simulink model "P702_NI_SoftECU"  (R2019a)
settings: Solver=ode1  StartTime=0.0  StopTime=Inf  FixedStep=0.001  RelTol=1e-3  EnableMultiTasking=on
PreLoadFcn:
  | run '.\VeriStand_BlockSet\NIVeriStandAddPaths.m'
undefined symbols (not defined in the file or in its folder): magnitude
libraries: simulink x83, simulink_extras x1
(part 18 of 76)

== system P702_NI_SoftECU/Input/ECM_DIESEL PCM PCM_HEV/PowertrainData_1_0x421 ==
  AirCondFluidHi_P_Actl : Constant  Commented=on  Value=0
  Bus_Sig : BusCreator  Inputs=12
  CoolantFanStepAct : Constant  Commented=on  Value=0
  ECMMILRequest : Constant  Commented=on  Value=0
  EngIdlShutDown_D_Stat : Constant  Commented=on  Value=0
  EngIdlShutDwnTxt_D_Rq : Constant  Commented=on  Value=0
  FUEL_ALCOHOL_PERCNT : Constant  Commented=on  Value=100.393700685
  FohEng_D_Rq : Constant  Commented=on  Value=2
  OilPressureWarning : Constant  Commented=on  Value=0
  TrnTotLss_Tq_Est : Constant  Commented=on  Value=0
  TrnTotTq_Rt_Est : Constant  Commented=on  Value=0
  VehVLimActv_B_Actl : Constant  Commented=on  Value=0
  VehVLimStat_D_Actl : Constant  Commented=on  Value=0
  PowertrainData_1_0x421 : Outport
  wires:
  Bus_Sig/1 -> PowertrainData_1_0x421/1  "PowertrainData_1_0x421"
  VehVLimActv_B_Actl/1 -> Bus_Sig/1  "VehVLimActv_B_Actl"
  VehVLimStat_D_Actl/1 -> Bus_Sig/2  "VehVLimStat_D_Actl"
  ECMMILRequest/1 -> Bus_Sig/3  "ECMMILRequest"
  FohEng_D_Rq/1 -> Bus_Sig/4  "FohEng_D_Rq"
  EngIdlShutDown_D_Stat/1 -> Bus_Sig/5  "EngIdlShutDown_D_Stat"
  CoolantFanStepAct/1 -> Bus_Sig/6  "CoolantFanStepAct"
  OilPressureWarning/1 -> Bus_Sig/7  "OilPressureWarning"
  EngIdlShutDwnTxt_D_Rq/1 -> Bus_Sig/8  "EngIdlShutDwnTxt_D_Rq"
  TrnTotLss_Tq_Est/1 -> Bus_Sig/9  "TrnTotLss_Tq_Est"
  TrnTotTq_Rt_Est/1 -> Bus_Sig/10  "TrnTotTq_Rt_Est"
  AirCondFluidHi_P_Actl/1 -> Bus_Sig/11  "AirCondFluidHi_P_Actl"
  FUEL_ALCOHOL_PERCNT/1 -> Bus_Sig/12  "FUEL_ALCOHOL_PERCNT"

== system P702_NI_SoftECU/Input/ECM_DIESEL PCM PCM_HEV/PowertrainData_2_0x42D ==
  ApedPos_Pc_ActlDiag : Constant  Commented=on  Value=0
  Bus_Sig : BusCreator  Inputs=11
  EngAirIn_Te_Actl : Constant  Commented=on  Value=-128
  EngClnt_Te_ActlDiag : Constant  Commented=on  Value=-40
  EngLoad_Pc_CalcDiag : Constant  Commented=on  Value=0
  EngMsgTxt_D_Rq : Constant  Commented=on  Value=0
  GrllShtrPos_B_Falt : Constant  Commented=on  Value=0
  GrllShtrPos_D_Cmd : Constant  Commented=on  Value=0
  IsaOffst_D_Stat : Constant  Commented=on  Value=0
  ObdWarmUp_B_Complt : Constant  Commented=on  Value=0
  SlMde_D_RqDsply : Constant  Commented=on  Value=0
  SlMde_D_Stat : Constant  Commented=on  Value=0
  PowertrainData_2_0x42D : Outport
  wires:
  Bus_Sig/1 -> PowertrainData_2_0x42D/1  "PowertrainData_2_0x42D"
  ObdWarmUp_B_Complt/1 -> Bus_Sig/1  "ObdWarmUp_B_Complt"
  EngMsgTxt_D_Rq/1 -> Bus_Sig/2  "EngMsgTxt_D_Rq"
  EngAirIn_Te_Actl/1 -> Bus_Sig/3  "EngAirIn_Te_Actl"
  ApedPos_Pc_ActlDiag/1 -> Bus_Sig/4  "ApedPos_Pc_ActlDiag"
  EngClnt_Te_ActlDiag/1 -> Bus_Sig/5  "EngClnt_Te_ActlDiag"
  EngLoad_Pc_CalcDiag/1 -> Bus_Sig/6  "EngLoad_Pc_CalcDiag"
  GrllShtrPos_D_Cmd/1 -> Bus_Sig/7  "GrllShtrPos_D_Cmd"
  GrllShtrPos_B_Falt/1 -> Bus_Sig/8  "GrllShtrPos_B_Falt"
  IsaOffst_D_Stat/1 -> Bus_Sig/9  "IsaOffst_D_Stat"
  SlMde_D_RqDsply/1 -> Bus_Sig/10  "SlMde_D_RqDsply"
  SlMde_D_Stat/1 -> Bus_Sig/11  "SlMde_D_Stat"

== system P702_NI_SoftECU/Input/ECM_DIESEL PCM PCM_HEV/PowertrainData_3_0x43E ==
  BattULoChrg_U_Cmd : Constant  Commented=on  Value=10.6
  Bus_Sig : BusCreator  Inputs=4
  ElLoadCtl_D_Rq : Constant  Commented=on  Value=0
  EngMnfld_P_Actl : Constant  Commented=on  Value=-206.8
  FuelPumpPwr_B_Rq : Constant  Commented=on  Value=0
  PowertrainData_3_0x43E : Outport
  wires:
  Bus_Sig/1 -> PowertrainData_3_0x43E/1  "PowertrainData_3_0x43E"
  BattULoChrg_U_Cmd/1 -> Bus_Sig/1  "BattULoChrg_U_Cmd"
  ElLoadCtl_D_Rq/1 -> Bus_Sig/2  "ElLoadCtl_D_Rq"
  FuelPumpPwr_B_Rq/1 -> Bus_Sig/3  "FuelPumpPwr_B_Rq"
  EngMnfld_P_Actl/1 -> Bus_Sig/4  "EngMnfld_P_Actl"

== system P702_NI_SoftECU/Input/ECM_DIESEL PCM PCM_HEV/PowertrainData_6_0x205 ==
  BrkTot_Tq_RqFapLc : Constant  Commented=on  Value=0
  Bus_Sig : BusCreator  Inputs=3
  FapLc_B_Err : S-Function  Priority=1  FunctionName=NIVeriStandIO  Parameters=width dtype portnum stime stype btype  SFunctionDeploymentMode=off  EnableBusSupport=off  mask(NI VeriStand Inport){portnum=1, width=1, stime=-1, dtype=auto, stype=auto, btype=1}
      mask prompts: portnum "Port number:"; width "Port dimensions (-1 for dynamically sized):"; stime "Sample time (-1 for inherited):"; dtype "Data type:"; stype "Signal type:"; btype "Block type:"
      mask help: Use this inport on any level of nested subsystems to allow NI VeriStand software to map signals to it.
      mask init:
      | NIVeriStandIO_init;
      settings: CopyFcn=NIVeriStand_MDL_functions('', 'IO_copy');  DeleteFcn=NIVeriStand_MDL_functions('', 'IO_delete');  MoveFcn=set_param(gcb, 'Mask', 'on');
      mask Callback portnum: NIVeriStand_MDL_functions('', 'IO_setportnum');
      mask TypeOptions dtype: auto | double | single | int8 | uint8 | int16 | uint16 | int32 | uint32 | boolean
      mask Callback dtype: NIVeriStand_MDL_functions('', 'IO_booleansignal');
      mask TypeOptions stype: auto | real | complex
      mask Display:
      | patch([-x x], [-y y], [.90980 .81960 .32156]);
      | plot([xrad -x x xrad], [yrad -y y yrad]);
      | fprintf('NI In%d', portnum);
  TrnAin_Pc_RqDrv : Constant  Commented=on  Value=0
  PowertrainData_6_0x205 : Outport
  wires:
  Bus_Sig/1 -> PowertrainData_6_0x205/1  "PowertrainData_6_0x205"
  BrkTot_Tq_RqFapLc/1 -> Bus_Sig/1  "BrkTot_Tq_RqFapLc"
  FapLc_B_Err/1 -> Bus_Sig/2  "FapLc_B_Err"
  TrnAin_Pc_RqDrv/1 -> Bus_Sig/3  "TrnAin_Pc_RqDrv"

== system P702_NI_SoftECU/Input/ECM_DIESEL PCM PCM_HEV/PowertrainData_7_0x41F ==
  Bus_Sig : BusCreator  Inputs=7
  EcoCochA_Pc_Dsply : Constant  Commented=on  Value=100.000035
  EcoCochCrus_Pc_Dsply : Constant  Commented=on  Value=100.000035
  EcoCochDecel_Pc_Dsply : Constant  Commented=on  Value=100.000035
  EcoCochIdlFuel_Pc_Dsply : Constant  Commented=on  Value=100.000035
  EcoCochInstNeg_B_Dsply : Constant  Commented=on  Value=0
  EcoCochInst_Pc_Dsply : Constant  Commented=on  Value=10
  EcoCochShif_Pc_Dsply : Constant  Commented=on  Value=100.000035
  PowertrainData_7_0x41F : Outport
  wires:
  Bus_Sig/1 -> PowertrainData_7_0x41F/1  "PowertrainData_7_0x41F"
  EcoCochA_Pc_Dsply/1 -> Bus_Sig/1  "EcoCochA_Pc_Dsply"
  EcoCochCrus_Pc_Dsply/1 -> Bus_Sig/2  "EcoCochCrus_Pc_Dsply"
  EcoCochDecel_Pc_Dsply/1 -> Bus_Sig/3  "EcoCochDecel_Pc_Dsply"
  EcoCochIdlFuel_Pc_Dsply/1 -> Bus_Sig/4  "EcoCochIdlFuel_Pc_Dsply"
  EcoCochShif_Pc_Dsply/1 -> Bus_Sig/5  "EcoCochShif_Pc_Dsply"
  EcoCochInst_Pc_Dsply/1 -> Bus_Sig/6  "EcoCochInst_Pc_Dsply"
  EcoCochInstNeg_B_Dsply/1 -> Bus_Sig/7  "EcoCochInstNeg_B_Dsply"

== system P702_NI_SoftECU/Input/ECM_DIESEL PCM PCM_HEV/PowertrainData_9_0x44C ==
  AutoTowActv_B_Stat : Constant  Commented=on  Value=0
  AutoTowAllw_D_StatMnu : Constant  Commented=on  Value=0
  Bus_Sig : BusCreator  Inputs=7
  GrossTrainWeight_M_Est : Constant  Commented=on  Value=25400
  TrailCtlPt_B_Falt : Constant  Commented=on  Value=0
  Veh_V_DsplyTrailCtlSet : Constant  Commented=on  Value=0
  WakeAlarm1_B_Typ : Constant  Commented=on  Value=0
  WakeAlarm1_T_Rq : Constant  Commented=on  Value=32767
  PowertrainData_9_0x44C : Outport
  wires:
  Bus_Sig/1 -> PowertrainData_9_0x44C/1  "PowertrainData_9_0x44C"
  GrossTrainWeight_M_Est/1 -> Bus_Sig/1  "GrossTrainWeight_M_Est"
  AutoTowAllw_D_StatMnu/1 -> Bus_Sig/2  "AutoTowAllw_D_StatMnu"
  AutoTowActv_B_Stat/1 -> Bus_Sig/3  "AutoTowActv_B_Stat"
  TrailCtlPt_B_Falt/1 -> Bus_Sig/4  "TrailCtlPt_B_Falt"
  Veh_V_DsplyTrailCtlSet/1 -> Bus_Sig/5  "Veh_V_DsplyTrailCtlSet"
  WakeAlarm1_T_Rq/1 -> Bus_Sig/6  "WakeAlarm1_T_Rq"
  WakeAlarm1_B_Typ/1 -> Bus_Sig/7  "WakeAlarm1_B_Typ"

== system P702_NI_SoftECU/Input/ECM_DIESEL PCM PCM_HEV/Powertrain_Data_4_0x424 ==
  BpedDrvMsgTxt_B_Dsply : Constant  Commented=on  Value=0
  Bus_Sig : BusCreator  Inputs=7
  FuelLvlWarn_D_ActlEng : Constant  Commented=on  Value=0
  FuelLvl_Pc_DsplyEng : Constant  Commented=on  Value=-5.217408
  FuelRange_L_DsplyEng : Constant  Commented=on  Value=0
  RearDiffOilTeWarn_B_Rq : Constant  Commented=on  Value=0
  RearDiffOil_Te_Actl : Constant  Commented=on  Value=37
  SelDrvMdePt_D_Stat : Constant  Commented=on  Value=0
  Powertrain_Data_4_0x424 : Outport
  wires:
  Bus_Sig/1 -> Powertrain_Data_4_0x424/1  "Powertrain_Data_4_0x424"
  BpedDrvMsgTxt_B_Dsply/1 -> Bus_Sig/1  "BpedDrvMsgTxt_B_Dsply"
  RearDiffOil_Te_Actl/1 -> Bus_Sig/2  "RearDiffOil_Te_Actl"
  RearDiffOilTeWarn_B_Rq/1 -> Bus_Sig/3  "RearDiffOilTeWarn_B_Rq"
  FuelLvlWarn_D_ActlEng/1 -> Bus_Sig/4  "FuelLvlWarn_D_ActlEng"
  SelDrvMdePt_D_Stat/1 -> Bus_Sig/5  "SelDrvMdePt_D_Stat"
  FuelRange_L_DsplyEng/1 -> Bus_Sig/6  "FuelRange_L_DsplyEng"
  FuelLvl_Pc_DsplyEng/1 -> Bus_Sig/7  "FuelLvl_Pc_DsplyEng"

== system P702_NI_SoftECU/Input/ECM_DIESEL PCM PCM_HEV/Powertrain_Data_5_0x43F ==
  Bus_Sig : BusCreator  Inputs=7
  FapLcActv_B_Stat : S-Function  Priority=1  FunctionName=NIVeriStandIO  Parameters=width dtype portnum stime stype btype  SFunctionDeploymentMode=off  EnableBusSupport=off  mask(NI VeriStand Inport){portnum=1, width=1, stime=-1, dtype=auto, stype=auto, btype=1}
      mask prompts: portnum "Port number:"; width "Port dimensions (-1 for dynamically sized):"; stime "Sample time (-1 for inherited):"; dtype "Data type:"; stype "Signal type:"; btype "Block type:"
      mask help: Use this inport on any level of nested subsystems to allow NI VeriStand software to map signals to it.
      mask init:
      | NIVeriStandIO_init;
      settings: CopyFcn=NIVeriStand_MDL_functions('', 'IO_copy');  DeleteFcn=NIVeriStand_MDL_functions('', 'IO_delete');  MoveFcn=set_param(gcb, 'Mask', 'on');
      mask Callback portnum: NIVeriStand_MDL_functions('', 'IO_setportnum');
      mask TypeOptions dtype: auto | double | single | int8 | uint8 | int16 | uint16 | int32 | uint32 | boolean
      mask Callback dtype: NIVeriStand_MDL_functions('', 'IO_booleansignal');
      mask TypeOptions stype: auto | real | complex
      mask Display:
      | patch([-x x], [-y y], [.90980 .81960 .32156]);
      | plot([xrad -x x xrad], [yrad -y y yrad]);
      | fprintf('NI In%d', portnum);
  FapLcInhbt_B_Rq : Constant  Commented=on  Value=0
  FapLcMaxGrdAbrt_B_Stat : S-Function  Priority=2  FunctionName=NIVeriStandIO  Parameters=width dtype portnum stime stype btype  SFunctionDeploymentMode=off  EnableBusSupport=off  mask(NI VeriStand Inport){portnum=2, width=1, stime=-1, dtype=auto, stype=auto, btype=1}
      mask prompts: portnum "Port number:"; width "Port dimensions (-1 for dynamically sized):"; stime "Sample time (-1 for inherited):"; dtype "Data type:"; stype "Signal type:"; btype "Block type:"
      mask help: Use this inport on any level of nested subsystems to allow NI VeriStand software to map signals to it.
      mask init:
      | NIVeriStandIO_init;
      settings: CopyFcn=NIVeriStand_MDL_functions('', 'IO_copy');  DeleteFcn=NIVeriStand_MDL_functions('', 'IO_delete');  MoveFcn=set_param(gcb, 'Mask', 'on');
      mask Callback portnum: NIVeriStand_MDL_functions('', 'IO_setportnum');
      mask TypeOptions dtype: auto | double | single | int8 | uint8 | int16 | uint16 | int32 | uint32 | boolean
      mask Callback dtype: NIVeriStand_MDL_functions('', 'IO_booleansignal');
      mask TypeOptions stype: auto | real | complex
      mask Display:
      | patch([-x x], [-y y], [.90980 .81960 .32156]);
      | plot([xrad -x x xrad], [yrad -y y yrad]);
      | fprintf('NI In%d', portnum);
  FapLcMaxGrdInhbt_B_Stat : S-Function  Priority=3  FunctionName=NIVeriStandIO  Parameters=width dtype portnum stime stype btype  SFunctionDeploymentMode=off  EnableBusSupport=off  mask(NI VeriStand Inport){portnum=3, width=1, stime=-1, dtype=auto, stype=auto, btype=1}
      mask prompts: portnum "Port number:"; width "Port dimensions (-1 for dynamically sized):"; stime "Sample time (-1 for inherited):"; dtype "Data type:"; stype "Signal type:"; btype "Block type:"
      mask help: Use this inport on any level of nested subsystems to allow NI VeriStand software to map signals to it.
      mask init:
      | NIVeriStandIO_init;
      settings: CopyFcn=NIVeriStand_MDL_functions('', 'IO_copy');  DeleteFcn=NIVeriStand_MDL_functions('', 'IO_delete');  MoveFcn=set_param(gcb, 'Mask', 'on');
      mask Callback portnum: NIVeriStand_MDL_functions('', 'IO_setportnum');
      mask TypeOptions dtype: auto | double | single | int8 | uint8 | int16 | uint16 | int32 | uint32 | boolean
      mask Callback dtype: NIVeriStand_MDL_functions('', 'IO_booleansignal');
      mask TypeOptions stype: auto | real | complex
      mask Display:
      | patch([-x x], [-y y], [.90980 .81960 .32156]);
      | plot([xrad -x x xrad], [yrad -y y yrad]);
      | fprintf('NI In%d', portnum);
  FapLcObstcl_B_Stat : S-Function  Priority=4  FunctionName=NIVeriStandIO  Parameters=width dtype portnum stime stype btype  SFunctionDeploymentMode=off  EnableBusSupport=off  mask(NI VeriStand Inport){portnum=4, width=1, stime=-1, dtype=auto, stype=auto, btype=1}
      mask prompts: portnum "Port number:"; width "Port dimensions (-1 for dynamically sized):"; stime "Sample time (-1 for inherited):"; dtype "Data type:"; stype "Signal type:"; btype "Block type:"
      mask help: Use this inport on any level of nested subsystems to allow NI VeriStand software to map signals to it.
      mask init:
      | NIVeriStandIO_init;
      settings: CopyFcn=NIVeriStand_MDL_functions('', 'IO_copy');  DeleteFcn=NIVeriStand_MDL_functions('', 'IO_delete');  MoveFcn=set_param(gcb, 'Mask', 'on');
      mask Callback portnum: NIVeriStand_MDL_functions('', 'IO_setportnum');
      mask TypeOptions dtype: auto | double | single | int8 | uint8 | int16 | uint16 | int32 | uint32 | boolean
      mask Callback dtype: NIVeriStand_MDL_functions('', 'IO_booleansignal');
      mask TypeOptions stype: auto | real | complex
      mask Display:
      | patch([-x x], [-y y], [.90980 .81960 .32156]);
      | plot([xrad -x x xrad], [yrad -y y yrad]);
      | fprintf('NI In%d', portnum);
  FapLcPrchgBrk_B_Rq : Constant  Commented=on  Value=0
  FapLcStopHold_B_Rq : Constant  Commented=on  Value=0
  Powertrain_Data_5_0x43F : Outport
  wires:
  Bus_Sig/1 -> Powertrain_Data_5_0x43F/1  "Powertrain_Data_5_0x43F"
  FapLcActv_B_Stat/1 -> Bus_Sig/1  "FapLcActv_B_Stat"
  FapLcMaxGrdAbrt_B_Stat/1 -> Bus_Sig/2  "FapLcMaxGrdAbrt_B_Stat"
  FapLcMaxGrdInhbt_B_Stat/1 -> Bus_Sig/3  "FapLcMaxGrdInhbt_B_Stat"
  FapLcObstcl_B_Stat/1 -> Bus_Sig/4  "FapLcObstcl_B_Stat"
  FapLcPrchgBrk_B_Rq/1 -> Bus_Sig/5  "FapLcPrchgBrk_B_Rq"
  FapLcStopHold_B_Rq/1 -> Bus_Sig/6  "FapLcStopHold_B_Rq"
  FapLcInhbt_B_Rq/1 -> Bus_Sig/7  "FapLcInhbt_B_Rq"

== system P702_NI_SoftECU/Input/ECM_DIESEL PCM PCM_HEV/Stop_Start_0x166 ==
  AutoStopPtDelta_I_Est : Constant  Commented=on  Value=-127
  Bus_Sig : BusCreator  Inputs=7
  HiElPwInhbt_B_Stat : Constant  Commented=on  Value=0
  OdoTripVerify_L_Actl : Constant  Commented=on  Value=0
  StopStrtDrvMde_D_Indic : Constant  Commented=on  Value=0
  StopStrtIODTxt_D_Rq : Constant  Commented=on  Value=0
  StopStrtMsgTxt_D_Rq : Constant  Commented=on  Value=0
  StopStrtStdby_D_Indic : Constant  Commented=on  Value=0
  Stop_Start_0x166 : Outport
  wires:
  Bus_Sig/1 -> Stop_Start_0x166/1  "Stop_Start_0x166"
  AutoStopPtDelta_I_Est/1 -> Bus_Sig/1  "AutoStopPtDelta_I_Est"
  HiElPwInhbt_B_Stat/1 -> Bus_Sig/2  "HiElPwInhbt_B_Stat"
  StopStrtDrvMde_D_Indic/1 -> Bus_Sig/3  "StopStrtDrvMde_D_Indic"
  StopStrtMsgTxt_D_Rq/1 -> Bus_Sig/4  "StopStrtMsgTxt_D_Rq"
  OdoTripVerify_L_Actl/1 -> Bus_Sig/5  "OdoTripVerify_L_Actl"
  StopStrtStdby_D_Indic/1 -> Bus_Sig/6  "StopStrtStdby_D_Indic"
  StopStrtIODTxt_D_Rq/1 -> Bus_Sig/7  "StopStrtIODTxt_D_Rq"

== system P702_NI_SoftECU/Input/ECM_DIESEL PCM PCM_HEV/TesterPhysicalResPCM_0x7E8 ==
  Bus_Sig : BusCreator  Inputs=1
  TesterPhysicalResPCM : Constant  Commented=on  Value=0
  TesterPhysicalResPCM_0x7E8 : Outport
  wires:
  Bus_Sig/1 -> TesterPhysicalResPCM_0x7E8/1  "TesterPhysicalResPCM_0x7E8"
  TesterPhysicalResPCM/1 -> Bus_Sig/1  "TesterPhysicalResPCM"

== system P702_NI_SoftECU/Input/ECM_DIESEL PCM PCM_HEV/TorqueDataEngFlags_0x200 ==
  Bus_Sig : BusCreator  Inputs=5
  PrplWhlTotTqRq_No_Cnt : Constant  Commented=on  Value=0
  PrplWhlTotTqRq_No_Cs : Constant  Commented=on  Value=0
  PrplWhlTot_Tq_LimMn : Constant  Commented=on  Value=-131072
  PrplWhlTot_Tq_Rq : S-Function  Priority=1  FunctionName=NIVeriStandIO  Parameters=width dtype portnum stime stype btype  SFunctionDeploymentMode=off  EnableBusSupport=off  mask(NI VeriStand Inport){portnum=1, width=1, stime=-1, dtype=auto, stype=auto, btype=1}
      mask prompts: portnum "Port number:"; width "Port dimensions (-1 for dynamically sized):"; stime "Sample time (-1 for inherited):"; dtype "Data type:"; stype "Signal type:"; btype "Block type:"
      mask help: Use this inport on any level of nested subsystems to allow NI VeriStand software to map signals to it.
      mask init:
      | NIVeriStandIO_init;
      settings: CopyFcn=NIVeriStand_MDL_functions('', 'IO_copy');  DeleteFcn=NIVeriStand_MDL_functions('', 'IO_delete');  MoveFcn=set_param(gcb, 'Mask', 'on');
      mask Callback portnum: NIVeriStand_MDL_functions('', 'IO_setportnum');
      mask TypeOptions dtype: auto | double | single | int8 | uint8 | int16 | uint16 | int32 | uint32 | boolean
      mask Callback dtype: NIVeriStand_MDL_functions('', 'IO_booleansignal');
      mask TypeOptions stype: auto | real | complex
      mask Display:
      | patch([-x x], [-y y], [.90980 .81960 .32156]);
      | plot([xrad -x x xrad], [yrad -y y yrad]);
      | fprintf('NI In%d', portnum);
  PtDrvMde_D_Stat : Constant  Commented=on  Value=0
  TorqueDataEngFlags_0x200 : Outport
  wires:
  Bus_Sig/1 -> TorqueDataEngFlags_0x200/1  "TorqueDataEngFlags_0x200"
  PrplWhlTot_Tq_LimMn/1 -> Bus_Sig/1  "PrplWhlTot_Tq_LimMn"
  PrplWhlTot_Tq_Rq/1 -> Bus_Sig/2  "PrplWhlTot_Tq_Rq"
  PtDrvMde_D_Stat/1 -> Bus_Sig/3  "PtDrvMde_D_Stat"
  PrplWhlTotTqRq_No_Cnt/1 -> Bus_Sig/4  "PrplWhlTotTqRq_No_Cnt"
  PrplWhlTotTqRq_No_Cs/1 -> Bus_Sig/5  "PrplWhlTotTqRq_No_Cs"

== system P702_NI_SoftECU/Input/ECM_DIESEL PCM PCM_HEV/TransGearData ==
  Bus_Sig : BusCreator  Inputs=5
  GboxOil_Te_Actl : Constant  Value=254
  GearLvrPos_D_Actl : S-Function  Priority=1  FunctionName=NIVeriStandIO  Parameters=width dtype portnum stime stype btype  SFunctionDeploymentMode=off  EnableBusSupport=off  mask(NI VeriStand Inport){portnum=1, width=1, stime=-1, dtype=auto, stype=auto, btype=1}
      mask prompts: portnum "Port number:"; width "Port dimensions (-1 for dynamically sized):"; stime "Sample time (-1 for inherited):"; dtype "Data type:"; stype "Signal type:"; btype "Block type:"
      mask help: Use this inport on any level of nested subsystems to allow NI VeriStand software to map signals to it.
      mask init:
      | NIVeriStandIO_init;
      settings: CopyFcn=NIVeriStand_MDL_functions('', 'IO_copy');  DeleteFcn=NIVeriStand_MDL_functions('', 'IO_delete');  MoveFcn=set_param(gcb, 'Mask', 'on');
      mask Callback portnum: NIVeriStand_MDL_functions('', 'IO_setportnum');
      mask TypeOptions dtype: auto | double | single | int8 | uint8 | int16 | uint16 | int32 | uint32 | boolean
      mask Callback dtype: NIVeriStand_MDL_functions('', 'IO_booleansignal');
      mask TypeOptions stype: auto | real | complex
      mask Display:
      | patch([-x x], [-y y], [.90980 .81960 .32156]);
      | plot([xrad -x x xrad], [yrad -y y yrad]);
      | fprintf('NI In%d', portnum);
  SelDrvMdeSwtch_D_Stat3 : Constant  Value=0
  TrnShifActv_B_Actl : Constant  Value=0
  TrnSrvcRqd_B_Rq : S-Function  Priority=2  FunctionName=NIVeriStandIO  Parameters=width dtype portnum stime stype btype  SFunctionDeploymentMode=off  EnableBusSupport=off  mask(NI VeriStand Inport){portnum=2, width=1, stime=-1, dtype=auto, stype=auto, btype=1}
      mask prompts: portnum "Port number:"; width "Port dimensions (-1 for dynamically sized):"; stime "Sample time (-1 for inherited):"; dtype "Data type:"; stype "Signal type:"; btype "Block type:"
      mask help: Use this inport on any level of nested subsystems to allow NI VeriStand software to map signals to it.
      mask init:
      | NIVeriStandIO_init;
      settings: CopyFcn=NIVeriStand_MDL_functions('', 'IO_copy');  DeleteFcn=NIVeriStand_MDL_functions('', 'IO_delete');  MoveFcn=set_param(gcb, 'Mask', 'on');
      mask Callback portnum: NIVeriStand_MDL_functions('', 'IO_setportnum');
      mask TypeOptions dtype: auto | double | single | int8 | uint8 | int16 | uint16 | int32 | uint32 | boolean
      mask Callback dtype: NIVeriStand_MDL_functions('', 'IO_booleansignal');
      mask TypeOptions stype: auto | real | complex
      mask Display:
      | patch([-x x], [-y y], [.90980 .81960 .32156]);
      | plot([xrad -x x xrad], [yrad -y y yrad]);
      | fprintf('NI In%d', portnum);
  TransGearData_230 : Outport
  wires:
  Bus_Sig/1 -> TransGearData_230/1  "TransGearData_230"
  GboxOil_Te_Actl/1 -> Bus_Sig/1  "GboxOil_Te_Actl"
  GearLvrPos_D_Actl/1 -> Bus_Sig/2  "GearLvrPos_D_Actl"
  SelDrvMdeSwtch_D_Stat3/1 -> Bus_Sig/3  "SelDrvMdeSwtch_D_Stat3"
  TrnShifActv_B_Actl/1 -> Bus_Sig/4  "TrnShifActv_B_Actl"
  TrnSrvcRqd_B_Rq/1 -> Bus_Sig/5  "TrnSrvcRqd_B_Rq"

== system P702_NI_SoftECU/Input/ECM_DIESEL PCM PCM_HEV/VehicleOperatingModes_0x167 ==
  Bus_Sig : BusCreator  Inputs=9
  ElPw_D_Stat : S-Function  Priority=3  FunctionName=NIVeriStandIO  Parameters=width dtype portnum stime stype btype  SFunctionDeploymentMode=off  EnableBusSupport=off  mask(NI VeriStand Inport){portnum=3, width=1, stime=-1, dtype=auto, stype=auto, btype=1}
      mask prompts: portnum "Port number:"; width "Port dimensions (-1 for dynamically sized):"; stime "Sample time (-1 for inherited):"; dtype "Data type:"; stype "Signal type:"; btype "Block type:"
      mask help: Use this inport on any level of nested subsystems to allow NI VeriStand software to map signals to it.
      mask init:
      | NIVeriStandIO_init;
      settings: CopyFcn=NIVeriStand_MDL_functions('', 'IO_copy');  DeleteFcn=NIVeriStand_MDL_functions('', 'IO_delete');  MoveFcn=set_param(gcb, 'Mask', 'on');
      mask Callback portnum: NIVeriStand_MDL_functions('', 'IO_setportnum');
      mask TypeOptions dtype: auto | double | single | int8 | uint8 | int16 | uint16 | int32 | uint32 | boolean
      mask Callback dtype: NIVeriStand_MDL_functions('', 'IO_booleansignal');
      mask TypeOptions stype: auto | real | complex
      mask Display:
      | patch([-x x], [-y y], [.90980 .81960 .32156]);
      | plot([xrad -x x xrad], [yrad -y y yrad]);
      | fprintf('NI In%d', portnum);
  ElPw_D_StatStrtStop : S-Function  Priority=5  FunctionName=NIVeriStandIO  Parameters=width dtype portnum stime stype btype  SFunctionDeploymentMode=off  EnableBusSupport=off  mask(NI VeriStand Inport){portnum=5, width=1, stime=-1, dtype=auto, stype=auto, btype=1}
      mask prompts: portnum "Port number:"; width "Port dimensions (-1 for dynamically sized):"; stime "Sample time (-1 for inherited):"; dtype "Data type:"; stype "Signal type:"; btype "Block type:"
      mask help: Use this inport on any level of nested subsystems to allow NI VeriStand software to map signals to it.
      mask init:
      | NIVeriStandIO_init;
      settings: CopyFcn=NIVeriStand_MDL_functions('', 'IO_copy');  DeleteFcn=NIVeriStand_MDL_functions('', 'IO_delete');  MoveFcn=set_param(gcb, 'Mask', 'on');
      mask Callback portnum: NIVeriStand_MDL_functions('', 'IO_setportnum');
      mask TypeOptions dtype: auto | double | single | int8 | uint8 | int16 | uint16 | int32 | uint32 | boolean
      mask Callback dtype: NIVeriStand_MDL_functions('', 'IO_booleansignal');
      mask TypeOptions stype: auto | real | complex
      mask Display:
      | patch([-x x], [-y y], [.90980 .81960 .32156]);
      | plot([xrad -x x xrad], [yrad -y y yrad]);
      | fprintf('NI In%d', portnum);
  Eng_D_Stat : S-Function  Priority=2  FunctionName=NIVeriStandIO  Parameters=width dtype portnum stime stype btype  SFunctionDeploymentMode=off  EnableBusSupport=off  mask(NI VeriStand Inport){portnum=2, width=1, stime=-1, dtype=auto, stype=auto, btype=1}
      mask prompts: portnum "Port number:"; width "Port dimensions (-1 for dynamically sized):"; stime "Sample time (-1 for inherited):"; dtype "Data type:"; stype "Signal type:"; btype "Block type:"
      mask help: Use this inport on any level of nested subsystems to allow NI VeriStand software to map signals to it.
      mask init:
      | NIVeriStandIO_init;
      settings: CopyFcn=NIVeriStand_MDL_functions('', 'IO_copy');  DeleteFcn=NIVeriStand_MDL_functions('', 'IO_delete');  MoveFcn=set_param(gcb, 'Mask', 'on');
      mask Callback portnum: NIVeriStand_MDL_functions('', 'IO_setportnum');
      mask TypeOptions dtype: auto | double | single | int8 | uint8 | int16 | uint16 | int32 | uint32 | boolean
      mask Callback dtype: NIVeriStand_MDL_functions('', 'IO_booleansignal');
      mask TypeOptions stype: auto | real | complex
      mask Display:
      | patch([-x x], [-y y], [.90980 .81960 .32156]);
      | plot([xrad -x x xrad], [yrad -y y yrad]);
      | fprintf('NI In%d', portnum);
  PlgActvArb_B_Actl : Constant  Commented=on
  PrplWhlRgenMn_Tq_Actl : Constant  Commented=on  Value=-16380
  PrplWhlTot2_Tq_Actl : S-Function  Priority=4  FunctionName=NIVeriStandIO  Parameters=width dtype portnum stime stype btype  SFunctionDeploymentMode=off  EnableBusSupport=off  mask(NI VeriStand Inport){portnum=4, width=1, stime=-1, dtype=auto, stype=auto, btype=1}
      mask prompts: portnum "Port number:"; width "Port dimensions (-1 for dynamically sized):"; stime "Sample time (-1 for inherited):"; dtype "Data type:"; stype "Signal type:"; btype "Block type:"
      mask help: Use this inport on any level of nested subsystems to allow NI VeriStand software to map signals to it.
      mask init:
      | NIVeriStandIO_init;
      settings: CopyFcn=NIVeriStand_MDL_functions('', 'IO_copy');  DeleteFcn=NIVeriStand_MDL_functions('', 'IO_delete');  MoveFcn=set_param(gcb, 'Mask', 'on');
      mask Callback portnum: NIVeriStand_MDL_functions('', 'IO_setportnum');
      mask TypeOptions dtype: auto | double | single | int8 | uint8 | int16 | uint16 | int32 | uint32 | boolean
      mask Callback dtype: NIVeriStand_MDL_functions('', 'IO_booleansignal');
      mask TypeOptions stype: auto | real | complex
      mask Display:
      | patch([-x x], [-y y], [.90980 .81960 .32156]);
      | plot([xrad -x x xrad], [yrad -y y yrad]);
      | fprintf('NI In%d', portnum);
  PwPckTq_D_Stat : S-Function  Priority=1  FunctionName=NIVeriStandIO  Parameters=width dtype portnum stime stype btype  SFunctionDeploymentMode=off  EnableBusSupport=off  mask(NI VeriStand Inport){portnum=1, width=1, stime=-1, dtype=auto, stype=auto, btype=1}
      mask prompts: portnum "Port number:"; width "Port dimensions (-1 for dynamically sized):"; stime "Sample time (-1 for inherited):"; dtype "Data type:"; stype "Signal type:"; btype "Block type:"
      mask help: Use this inport on any level of nested subsystems to allow NI VeriStand software to map signals to it.
      mask init:
      | NIVeriStandIO_init;
      settings: CopyFcn=NIVeriStand_MDL_functions('', 'IO_copy');  DeleteFcn=NIVeriStand_MDL_functions('', 'IO_delete');  MoveFcn=set_param(gcb, 'Mask', 'on');
      mask Callback portnum: NIVeriStand_MDL_functions('', 'IO_setportnum');
      mask TypeOptions dtype: auto | double | single | int8 | uint8 | int16 | uint16 | int32 | uint32 | boolean
      mask Callback dtype: NIVeriStand_MDL_functions('', 'IO_booleansignal');
      mask TypeOptions stype: auto | real | complex
      mask Display:
      | patch([-x x], [-y y], [.90980 .81960 .32156]);
      | plot([xrad -x x xrad], [yrad -y y yrad]);
      | fprintf('NI In%d', portnum);
  TrnAinTq_D_Qf : Constant  Commented=on  Value=0
  TrnAin_Tq_Actl : Constant  Commented=on  Value=-500
  VehicleOperatingModes_0x167 : Outport
  wires:
  Bus_Sig/1 -> VehicleOperatingModes_0x167/1  "VehicleOperatingModes_0x167"
  Eng_D_Stat/1 -> Bus_Sig/1  "Eng_D_Stat"
  PwPckTq_D_Stat/1 -> Bus_Sig/2  "PwPckTq_D_Stat"
  ElPw_D_Stat/1 -> Bus_Sig/3  "ElPw_D_Stat"
  PlgActvArb_B_Actl/1 -> Bus_Sig/4  "PlgActvArb_B_Actl"
  PrplWhlTot2_Tq_Actl/1 -> Bus_Sig/5  "PrplWhlTot2_Tq_Actl"
  ElPw_D_StatStrtStop/1 -> Bus_Sig/6  "ElPw_D_StatStrtStop"
  PrplWhlRgenMn_Tq_Actl/1 -> Bus_Sig/7  "PrplWhlRgenMn_Tq_Actl"
  TrnAinTq_D_Qf/1 -> Bus_Sig/8  "TrnAinTq_D_Qf"
  TrnAin_Tq_Actl/1 -> Bus_Sig/9  "TrnAin_Tq_Actl"

== system P702_NI_SoftECU/Input/GWM-SCCM//PDB//RCM//GSM/GSM ==
  Enable : EnablePort
  Bus Creator : BusCreator  Inputs=2
  Gear_Shift_by_Wire_2_FD1 : Subsystem
  Gear_Shift_by_Wire_FD1 : Subsystem
  GSM_Signals : Outport
  wires:
  Bus Creator/1 -> GSM_Signals/1
  Gear_Shift_by_Wire_2_FD1/1(Gear_Shift_by_Wire_2_FD1_168) -> Bus Creator/1
  Gear_Shift_by_Wire_FD1/1(Gear_Shift_by_Wire_FD1_5A) -> Bus Creator/2

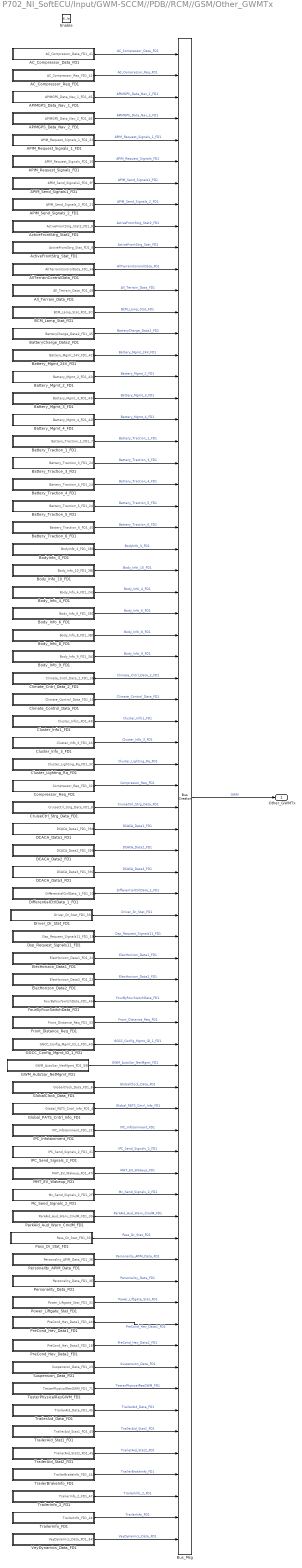
== system P702_NI_SoftECU/Input/GWM-SCCM//PDB//RCM//GSM/Other_GWMTx ==
  Enable : EnablePort
  AC_Compressor_Data_FD1 : Subsystem
  AC_Compressor_Req_FD1 : Subsystem
  APIMGPS_Data_Nav_1_FD1 : Subsystem
  APIMGPS_Data_Nav_2_FD1 : Subsystem
  APIM_Request_Signals_1_FD1 : Subsystem
  APIM_Request_Signals_FD1 : Subsystem
  APIM_Send_Signals1_FD1 : Subsystem
  APIM_Send_Signals_2_FD1 : Subsystem
  ActiveFrontStrg_Stat2_FD1 : Subsystem
  ActiveFrontStrg_Stat_FD1 : Subsystem
  AllTerrainControlData_FD1 : Subsystem
  All_Terrain_Data_FD1 : Subsystem
  BCM_Lamp_Stat_FD1 : Subsystem
  BatteryCharge_Data2_FD1 : Subsystem
  Battery_Mgmt_24V_FD1 : Subsystem
  Battery_Mgmt_2_FD1 : Subsystem
  Battery_Mgmt_3_FD1 : Subsystem
  Battery_Mgmt_4_FD1 : Subsystem
  Battery_Traction_1_FD1 : Subsystem
  Battery_Traction_3_FD1 : Subsystem
  Battery_Traction_4_FD1 : Subsystem
  Battery_Traction_5_FD1 : Subsystem
  Battery_Traction_6_FD1 : Subsystem
  BodyInfo_3_FD1 : Subsystem
  Body_Info_10_FD1 : Subsystem
  Body_Info_4_FD1 : Subsystem
  Body_Info_6_FD1 : Subsystem
  Body_Info_8_FD1 : Subsystem
  Body_Info_9_FD1 : Subsystem
  Bus_Msg : BusCreator  Inputs=70
  Climate_Cntrl_Data_2_FD1 : Subsystem
  Climate_Control_Data_FD1 : Subsystem
  Cluster_Info1_FD1 : Subsystem
  Cluster_Info_3_FD1 : Subsystem
  Cluster_Lighting_Rq_FD1 : Subsystem
  Compressor_Req_FD1 : Subsystem
  CruiseCtrl_Strg_Data_FD1 : Subsystem
  DCACA_Data1_FD1 : Subsystem
  DCACA_Data2_FD1 : Subsystem
  DCACA_Data3_FD1 : Subsystem
  DifferentialCtrlData_1_FD1 : Subsystem
  Driver_Dr_Stat_FD1 : Subsystem
  Dsp_Request_Signals11_FD1 : Subsystem
  ElecHorizon_Data1_FD1 : Subsystem
  ElecHorizon_Data2_FD1 : Subsystem
  FourByFourSwitchData_FD1 : Subsystem
  Front_Distance_Req_FD1 : Subsystem
  GGCC_Config_Mgmt_ID_1_FD1 : Subsystem
  GWM_AutoSar_NetMgmt_FD1 : Subsystem
  GlobalClock_Data_FD1 : Subsystem
  Global_PATS_Cntrl_Info_FD1 : Subsystem
  IPC_Infotainment_FD1 : Subsystem
  IPC_Send_Signals_2_FD1 : Subsystem
  MHT_EV_Wakeup_FD1 : Subsystem
  Mc_Send_Signals_2_FD1 : Subsystem
  ParkAid_Aud_Warn_CmdM_FD1 : Subsystem
  Pass_Dr_Stat_FD1 : Subsystem
  Personality_APIM_Data_FD1 : Subsystem
  Personality_Data_FD1 : Subsystem
  Power_Liftgate_Stat_FD1 : Subsystem
  PreCond_Hev_Data1_FD1 : Subsystem
  PreCond_Hev_Data2_FD1 : Subsystem
  Suspension_Data_FD1 : Subsystem
  TesterPhysicalResGWM_FD1 : Subsystem
  TrailerAid_Data_FD1 : Subsystem
  TrailerAid_Stat1_FD1 : Subsystem
  TrailerAid_Stat2_FD1 : Subsystem
  TrailerBrakeInfo_FD1 : Subsystem
  TrailerInfo_2_FD1 : Subsystem
  TrailerInfo_FD1 : Subsystem
  VeyDynamics_Data_FD1 : Subsystem
  Other_GWMTx : Outport
  wires:
  Bus_Msg/1 -> Other_GWMTx/1  "GWM"
  AC_Compressor_Data_FD1/1(AC_Compressor_Data_FD1_411) -> Bus_Msg/1  "AC_Compressor_Data_FD1"
  AC_Compressor_Req_FD1/1(AC_Compressor_Req_FD1_410) -> Bus_Msg/2  "AC_Compressor_Req_FD1"
  APIMGPS_Data_Nav_1_FD1/1(APIMGPS_Data_Nav_1_FD1_462) -> Bus_Msg/3  "APIMGPS_Data_Nav_1_FD1"
  APIMGPS_Data_Nav_2_FD1/1(APIMGPS_Data_Nav_2_FD1_463) -> Bus_Msg/4  "APIMGPS_Data_Nav_2_FD1"
  APIM_Request_Signals_1_FD1/1(APIM_Request_Signals_1_FD1_227) -> Bus_Msg/5  "APIM_Request_Signals_1_FD1"
  APIM_Request_Signals_FD1/1(APIM_Request_Signals_FD1_105) -> Bus_Msg/6  "APIM_Request_Signals_FD1"
  APIM_Send_Signals1_FD1/1(APIM_Send_Signals1_FD1_3F1) -> Bus_Msg/7  "APIM_Send_Signals1_FD1"
  APIM_Send_Signals_2_FD1/1(APIM_Send_Signals_2_FD1_215) -> Bus_Msg/8  "APIM_Send_Signals_2_FD1"
  ActiveFrontStrg_Stat2_FD1/1(ActiveFrontStrg_Stat2_FD1_8A) -> Bus_Msg/9  "ActiveFrontStrg_Stat2_FD1"
  ActiveFrontStrg_Stat_FD1/1(ActiveFrontStrg_Stat_FD1_89) -> Bus_Msg/10  "ActiveFrontStrg_Stat_FD1"
  AllTerrainControlData_FD1/1(AllTerrainControlData_FD1_461) -> Bus_Msg/11  "AllTerrainControlData_FD1"
  All_Terrain_Data_FD1/1(All_Terrain_Data_FD1_481) -> Bus_Msg/12  "All_Terrain_Data_FD1"
  BCM_Lamp_Stat_FD1/1(BCM_Lamp_Stat_FD1_3C3) -> Bus_Msg/13  "BCM_Lamp_Stat_FD1"
  BatteryCharge_Data2_FD1/1(BatteryCharge_Data2_FD1_45E) -> Bus_Msg/14  "BatteryCharge_Data2_FD1"
  Battery_Mgmt_24V_FD1/1(Battery_Mgmt_24V_FD1_42E) -> Bus_Msg/15  "Battery_Mgmt_24V_FD1"
  Battery_Mgmt_2_FD1/1(Battery_Mgmt_2_FD1_42C) -> Bus_Msg/16  "Battery_Mgmt_2_FD1"
  Battery_Mgmt_3_FD1/1(Battery_Mgmt_3_FD1_43C) -> Bus_Msg/17  "Battery_Mgmt_3_FD1"
  Battery_Mgmt_4_FD1/1(Battery_Mgmt_4_FD1_42B) -> Bus_Msg/18  "Battery_Mgmt_4_FD1"
  Battery_Traction_1_FD1/1(Battery_Traction_1_FD1_7A) -> Bus_Msg/19  "Battery_Traction_1_FD1"
  Battery_Traction_3_FD1/1(Battery_Traction_3_FD1_24B) -> Bus_Msg/20  "Battery_Traction_3_FD1"
  Battery_Traction_4_FD1/1(Battery_Traction_4_FD1_24C) -> Bus_Msg/21  "Battery_Traction_4_FD1"
  Battery_Traction_5_FD1/1(Battery_Traction_5_FD1_24D) -> Bus_Msg/22  "Battery_Traction_5_FD1"
  Battery_Traction_6_FD1/1(Battery_Traction_6_FD1_458) -> Bus_Msg/23  "Battery_Traction_6_FD1"
  BodyInfo_3_FD1/1(BodyInfo_3_FD1_3B3) -> Bus_Msg/24  "BodyInfo_3_FD1"
  Body_Info_10_FD1/1(Body_Info_10_FD1_3BA) -> Bus_Msg/25  "Body_Info_10_FD1"
  Body_Info_4_FD1/1(Body_Info_4_FD1_242) -> Bus_Msg/26  "Body_Info_4_FD1"
  Body_Info_6_FD1/1(Body_Info_6_FD1_38D) -> Bus_Msg/27  "Body_Info_6_FD1"
  Body_Info_8_FD1/1(Body_Info_8_FD1_3B9) -> Bus_Msg/28  "Body_Info_8_FD1"
  Body_Info_9_FD1/1(Body_Info_9_FD1_3A3) -> Bus_Msg/29  "Body_Info_9_FD1"
  Climate_Cntrl_Data_2_FD1/1(Climate_Cntrl_Data_2_FD1_35E) -> Bus_Msg/30  "Climate_Cntrl_Data_2_FD1"
  Climate_Control_Data_FD1/1(Climate_Control_Data_FD1_41A) -> Bus_Msg/31  "Climate_Control_Data_FD1"
  Cluster_Info1_FD1/1(Cluster_Info1_FD1_430) -> Bus_Msg/32  "Cluster_Info1_FD1"
  Cluster_Info_3_FD1/1(Cluster_Info_3_FD1_434) -> Bus_Msg/33  "Cluster_Info_3_FD1"
  Cluster_Lighting_Rq_FD1/1(Cluster_Lighting_Rq_FD1_3C8) -> Bus_Msg/34  "Cluster_Lighting_Rq_FD1"
  Compressor_Req_FD1/1(Compressor_Req_FD1_326) -> Bus_Msg/35  "Compressor_Req_FD1"
  CruiseCtrl_Strg_Data_FD1/1(CruiseCtrl_Strg_Data_FD1_8B) -> Bus_Msg/36  "CruiseCtrl_Strg_Data_FD1"
  DCACA_Data1_FD1/1(DCACA_Data1_FD1_39A) -> Bus_Msg/37  "DCACA_Data1_FD1"
  DCACA_Data2_FD1/1(DCACA_Data2_FD1_39B) -> Bus_Msg/38  "DCACA_Data2_FD1"
  DCACA_Data3_FD1/1(DCACA_Data3_FD1_39C) -> Bus_Msg/39  "DCACA_Data3_FD1"
  DifferentialCtrlData_1_FD1/1(DifferentialCtrlData_1_FD1_206) -> Bus_Msg/40  "DifferentialCtrlData_1_FD1"
  Driver_Dr_Stat_FD1/1(Driver_Dr_Stat_FD1_332) -> Bus_Msg/41  "Driver_Dr_Stat_FD1"
  Dsp_Request_Signals11_FD1/1(Dsp_Request_Signals11_FD1_192) -> Bus_Msg/42  "Dsp_Request_Signals11_FD1"
  ElecHorizon_Data1_FD1/1(ElecHorizon_Data1_FD1_22E) -> Bus_Msg/43  "ElecHorizon_Data1_FD1"
  ElecHorizon_Data2_FD1/1(ElecHorizon_Data2_FD1_22F) -> Bus_Msg/44  "ElecHorizon_Data2_FD1"
  FourByFourSwitchData_FD1/1(FourByFourSwitchData_FD1_460) -> Bus_Msg/45  "FourByFourSwitchData_FD1"
  Front_Distance_Req_FD1/1(Front_Distance_Req_FD1_339) -> Bus_Msg/46  "Front_Distance_Req_FD1"
  GGCC_Config_Mgmt_ID_1_FD1/1(GGCC_Config_Mgmt_ID_1_FD1_40A) -> Bus_Msg/47  "GGCC_Config_Mgmt_ID_1_FD1"
  GWM_AutoSar_NetMgmt_FD1/1(GWM_AutoSar_NetMgmt_FD1_59E) -> Bus_Msg/48  "GWM_AutoSar_NetMgmt_FD1"
  GlobalClock_Data_FD1/1(GlobalClock_Data_FD1_84) -> Bus_Msg/49  "GlobalClock_Data_FD1"
  Global_PATS_Cntrl_Info_FD1/1(Global_PATS_Cntrl_Info_FD1_41) -> Bus_Msg/50  "Global_PATS_Cntrl_Info_FD1"
  IPC_Send_Signals_2_FD1/1(IPC_Send_Signals_2_FD1_318) -> Bus_Msg/52  "IPC_Send_Signals_2_FD1"
  MHT_EV_Wakeup_FD1/1(MHT_EV_Wakeup_FD1_478) -> Bus_Msg/53  "MHT_EV_Wakeup_FD1"
  Mc_Send_Signals_2_FD1/1(Mc_Send_Signals_2_FD1_2FD) -> Bus_Msg/54  "Mc_Send_Signals_2_FD1"
  ParkAid_Aud_Warn_CmdM_FD1/1(ParkAid_Aud_Warn_CmdM_FD1_30A) -> Bus_Msg/55  "ParkAid_Aud_Warn_CmdM_FD1"
  Pass_Dr_Stat_FD1/1(Pass_Dr_Stat_FD1_333) -> Bus_Msg/56  "Pass_Dr_Stat_FD1"
  Personality_APIM_Data_FD1/1(Personality_APIM_Data_FD1_3E2) -> Bus_Msg/57  "Personality_APIM_Data_FD1"
  Personality_Data_FD1/1(Personality_Data_FD1_3E0) -> Bus_Msg/58  "Personality_Data_FD1"
  Power_Liftgate_Stat_FD1/1(Power_Liftgate_Stat_FD1_313) -> Bus_Msg/59  "Power_Liftgate_Stat_FD1"
  PreCond_Hev_Data1_FD1/1(PreCond_Hev_Data1_FD1_440) -> Bus_Msg/60  "PreCond_Hev_Data1_FD1"
  PreCond_Hev_Data2_FD1/1(PreCond_Hev_Data2_FD1_185) -> Bus_Msg/61  "PreCond_Hev_Data2_FD1"
  Suspension_Data_FD1/1(Suspension_Data_FD1_23A) -> Bus_Msg/62  "Suspension_Data_FD1"
  TesterPhysicalResGWM_FD1/1(TesterPhysicalResGWM_FD1_71E) -> Bus_Msg/63  "TesterPhysicalResGWM_FD1"
  TrailerAid_Data_FD1/1(TrailerAid_Data_FD1_45A) -> Bus_Msg/64  "TrailerAid_Data_FD1"
  TrailerAid_Stat1_FD1/1(TrailerAid_Stat1_FD1_452) -> Bus_Msg/65  "TrailerAid_Stat1_FD1"
  TrailerAid_Stat2_FD1/1(TrailerAid_Stat2_FD1_457) -> Bus_Msg/66  "TrailerAid_Stat2_FD1"
  TrailerBrakeInfo_FD1/1(TrailerBrakeInfo_FD1_445) -> Bus_Msg/67  "TrailerBrakeInfo_FD1"
  TrailerInfo_2_FD1/1(TrailerInfo_2_FD1_47A) -> Bus_Msg/68  "TrailerInfo_2_FD1"
  TrailerInfo_FD1/1(TrailerInfo_FD1_443) -> Bus_Msg/69  "TrailerInfo_FD1"
  VeyDynamics_Data_FD1/1(VeyDynamics_Data_FD1_345) -> Bus_Msg/70  "VeyDynamics_Data_FD1"
  IPC_Infotainment_FD1/1(IPC_Infotainment_FD1_225) -> Bus_Msg/51  "IPC_Infotainment_FD1"

== system P702_NI_SoftECU/Input/GWM-SCCM//PDB//RCM//GSM/RCM ==
  Enable : EnablePort
  Bus Creator : BusCreator  Inputs=2
  RCMSerialNumber_FD1 : Subsystem
  RCMStatusMessage2_FD1 : Subsystem
  RCM_Signals : Outport
  wires:
  RCMStatusMessage2_FD1/1(RCMStatusMessage2_FD1_4C) -> Bus Creator/1
  Bus Creator/1 -> RCM_Signals/1
  RCMSerialNumber_FD1/1(RCMSerialNumber_FD1_454) -> Bus Creator/2

== system P702_NI_SoftECU/Input/GWM-SCCM//PDB//RCM//GSM/SCCM ==
  Enable : EnablePort
  Bus Creator : BusCreator  Inputs=2
  Steering_Data_FD1 : Subsystem
  Steering_Wheel_Data2_FD1 : Subsystem
  SCCM_Signals : Outport
  wires:
  Bus Creator/1 -> SCCM_Signals/1
  Steering_Data_FD1/1(Steering_Data_FD1_83) -> Bus Creator/1
  Steering_Wheel_Data2_FD1/1(Steering_Wheel_Data2_FD1_81) -> Bus Creator/2

== system P702_NI_SoftECU/Input/GWM-SCCM//PDB//RCM//GSM/Tester//AutoSar ==
  Enable : EnablePort
  Bus_Msg : BusCreator  Inputs=2
  GWM_AutoSar_NetMgmt_FD1 : Subsystem
  TesterPhysicalResGWM_FD1 : Subsystem
  Tester/AutoSar : Outport
  wires:
  Bus_Msg/1 -> Tester/AutoSar/1  "GWM"
  GWM_AutoSar_NetMgmt_FD1/1(GWM_AutoSar_NetMgmt_FD1_59E) -> Bus_Msg/1  "GWM_AutoSar_NetMgmt_FD1"
  TesterPhysicalResGWM_FD1/1(TesterPhysicalResGWM_FD1_71E) -> Bus_Msg/2  "TesterPhysicalResGWM_FD1"
